simulink model "simfile"  (R2024a)
settings: Solver=VariableStepAuto  StartTime=0.0  StopTime=Sim_time  RelTol=1e-3
values from neighbouring files (symbols this model uses):
  Cn = 2.3 * 60 * 60    (= 8280)    [mscript.m]
  I = 2.3    [mscript.m]
  OCV = Data(:, 2)    [mscript.m]
  R_Charge = Data(:, 3)    [mscript.m]
  R_Discharge = Data(:,4)    [mscript.m]
  SOC = Data(:, 1)    [mscript.m]
settings Model: Creator=admin  LastModifiedBy=admin

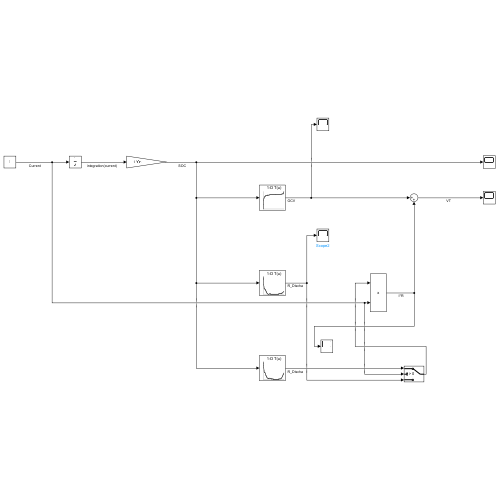
[thumbnail: Simulink's stored preview of the top-level diagram]
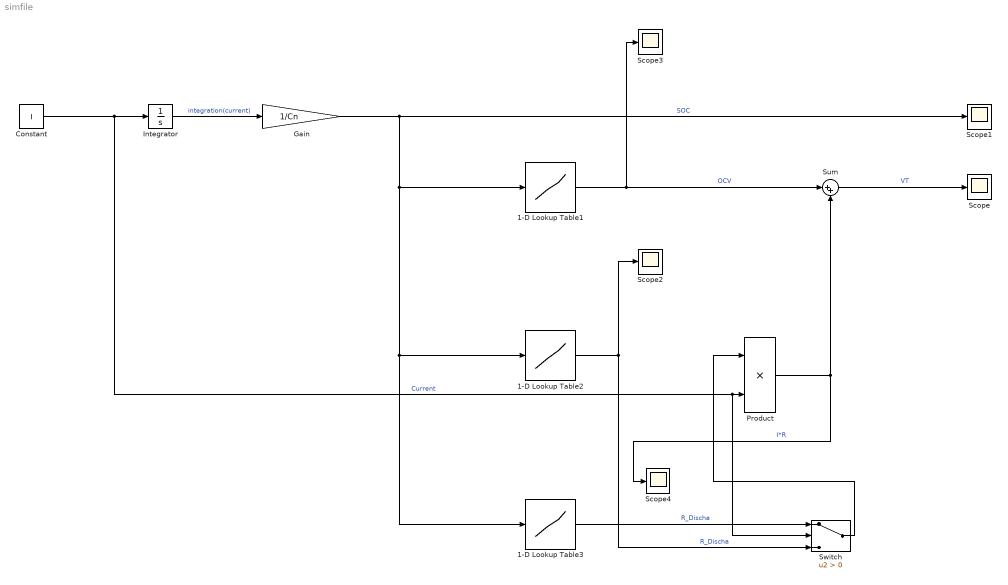
== system simfile ==
  1-D Lookup Table1 : Lookup_n-D  NumberOfTableDimensions=1  BreakpointsForDimension1=SOC  Table=OCV  InternalRulePriority=Speed  RndMeth=Simplest
  1-D Lookup Table2 : Lookup_n-D  NumberOfTableDimensions=1  BreakpointsForDimension1=SOC  Table=R_Discharge  InternalRulePriority=Speed  RndMeth=Simplest
  1-D Lookup Table3 : Lookup_n-D  NumberOfTableDimensions=1  BreakpointsForDimension1=SOC  Table=R_Charge  InternalRulePriority=Speed  RndMeth=Simplest
  Constant : Constant  Value=I
  Gain : Gain  Gain=1/Cn
  Integrator : Integrator
  Product : Product
  Scope{,1..4} (5 alike) : Scope
  Sum : Sum  Inputs=|++
  Switch : Switch  Criteria=u2 > Threshold  SaturateOnIntegerOverflow=off  InputSameDT=off
  wires:
  Constant/1 -> Switch/2, Product/2, Integrator/1  "Current"
  Integrator/1 -> Gain/1  "integration(current)"
  Gain/1 -> Scope1/1, 1-D Lookup Table3/1, 1-D Lookup Table2/1, 1-D Lookup Table1/1  "SOC"
  1-D Lookup Table2/1 -> Switch/3, Scope2/1  "R_Discha"
  1-D Lookup Table1/1 -> Scope3/1, Sum/1  "OCV"
  Product/1 -> Scope4/1, Sum/2  "I*R"
  Sum/1 -> Scope/1  "VT"
  Switch/1 -> Product/1
  1-D Lookup Table3/1 -> Switch/1  "R_Discha"
